simulink model "PID_Attitude_ver7_5"  (R2022a)
settings: Solver=FixedStepDiscrete  StartTime=0.0  StopTime=0.1  RelTol=1e-3
libraries: hdlsllib x1
settings Model: DataTypeOverride=Off  Creator=space  LastModifiedBy=space
settings OptimizationCC: BlockReduction=off  ConditionallyExecuteInputs=off  DefaultParameterBehavior=Inlined  InheritOutputTypeSmallerThanSingle=on
settings DebuggingCC: AlgebraicLoopMsg=error  SingleTaskRateTransMsg=error
settings HardwareCC: ProdBitPerPointer=32  ProdBitPerSizeT=32  ProdBitPerPtrDiffT=32  ProdLargestAtomicFloat=None  ProdIntDivRoundTo=Undefined  ProdEndianess=Unspecified  ProdWordSize=32  ProdHWDeviceType=ASIC/FPGA->ASIC/FPGA  TargetBitPerPointer=64  TargetBitPerSizeT=64  TargetBitPerPtrDiffT=64  TargetLongLongMode=on  TargetIntDivRoundTo=Zero  TargetEndianess=LittleEndian  TargetWordSize=64  TargetHWDeviceType=Custom Processor->MATLAB Host Computer  ProdEqTarget=off

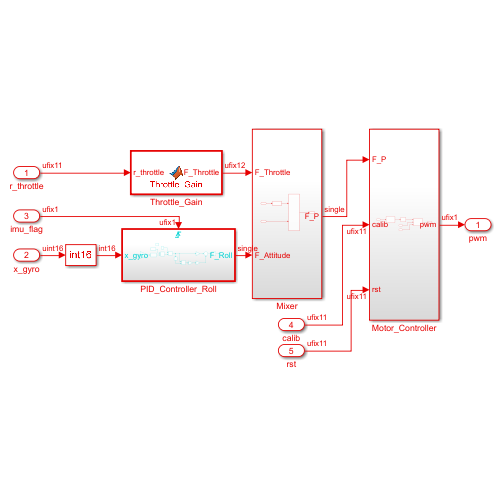
[thumbnail: Simulink's stored preview of the top-level diagram]
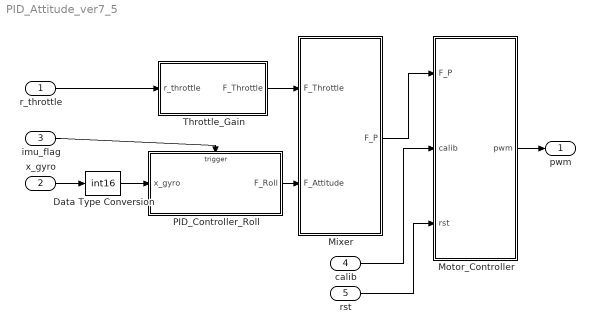
== system PID_Attitude_ver7_5 ==
  r_throttle : Inport  OutDataTypeStr=fixdt(0,11,0)
  x_gyro : Inport  Port=2  OutDataTypeStr=uint16
  imu_flag : Inport  Port=3  OutDataTypeStr=fixdt(0,1,0)
  calib : Inport  Port=4  OutDataTypeStr=fixdt(0,11,0)
  rst : Inport  Port=5  OutDataTypeStr=fixdt(0,11,0)
  Data Type Conversion : DataTypeConversion  OutDataTypeStr=int16  SaturateOnIntegerOverflow=off  RndMeth=Floor
  Mixer : Subsystem
  Motor_Controller : Subsystem
  PID_Controller_Roll : Subsystem
  Throttle_Gain : MATLAB Function  TreatAsAtomicUnit=on
  pwm : Outport  VectorParamsAs1DForOutWhenUnconnected=off
  wires:
  imu_flag/1 -> PID_Controller_Roll/Trigger
  Mixer/1(F_P) -> Motor_Controller/1(F_P)
  Motor_Controller/1(pwm) -> pwm/1
  rst/1 -> Motor_Controller/3(rst)
  r_throttle/1 -> Throttle_Gain/1(r_throttle)
  PID_Controller_Roll/1(F_Roll) -> Mixer/2(F_Attitude)
  Throttle_Gain/1(F_Throttle) -> Mixer/1(F_Throttle)
  x_gyro/1 -> Data Type Conversion/1
  Data Type Conversion/1 -> PID_Controller_Roll/1(x_gyro)
  calib/1 -> Motor_Controller/2(calib)

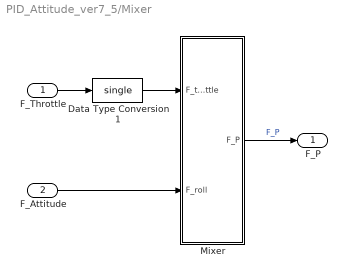
== system PID_Attitude_ver7_5/Mixer ==
  F_Throttle : Inport
  F_Attitude : Inport  Port=2
  Data Type Conversion1 : DataTypeConversion  OutDataTypeStr=single  SaturateOnIntegerOverflow=off  RndMeth=Floor
  Mixer : MATLAB Function  TreatAsAtomicUnit=on
  F_P : Outport
  wires:
  F_Throttle/1 -> Data Type Conversion1/1
  Mixer/1(F_P) -> F_P/1  "F_P"
  Data Type Conversion1/1 -> Mixer/1(F_throttle)
  F_Attitude/1 -> Mixer/2(F_roll)

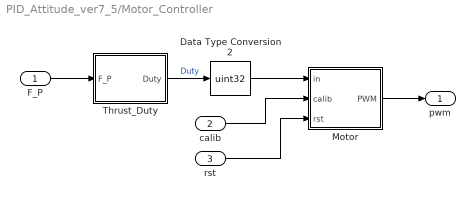
== system PID_Attitude_ver7_5/Motor_Controller ==
  F_P : Inport
  calib : Inport  Port=2  OutDataTypeStr=fixdt(0,11,0)
  rst : Inport  Port=3  OutDataTypeStr=fixdt(0,11,0)
  Data Type Conversion2 : DataTypeConversion  OutDataTypeStr=uint32  SaturateOnIntegerOverflow=off  RndMeth=Floor
  Motor : Subsystem
  Thrust_Duty : MATLAB Function  TreatAsAtomicUnit=on
  pwm : Outport
  wires:
  Thrust_Duty/1(Duty) -> Data Type Conversion2/1  "Duty"
  F_P/1 -> Thrust_Duty/1(F_P)
  Data Type Conversion2/1 -> Motor/1(in)
  calib/1 -> Motor/2(calib)
  rst/1 -> Motor/3(rst)
  Motor/1(PWM) -> pwm/1

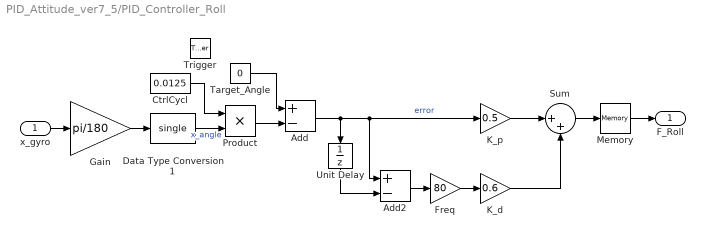
== system PID_Attitude_ver7_5/PID_Controller_Roll ==
  x_gyro : Inport
  Trigger : TriggerPort  VariantControl=(inherit)  PortDimensions=1
  Add : Sum  Inputs=+-
  Add2 : Sum  Inputs=+-
  CtrlCycl : Constant  Value=0.0125  VectorParams1D=off  OutDataTypeStr=single  SampleTime=-1
  Data Type Conversion1 : DataTypeConversion  OutDataTypeStr=single  SaturateOnIntegerOverflow=off  RndMeth=Floor
  Freq : Gain  Gain=80
  Gain : Gain  Gain=pi/180
  K_d : Gain  Gain=0.6
  K_p : Gain  Gain=0.5
  Memory : Memory  InheritSampleTime=on
  Product : Product
  Sum : Sum  Inputs=|++
  Target_Angle : Constant  Value=0  VectorParams1D=off  OutDataTypeStr=single  SampleTime=-1
  Unit Delay : UnitDelay  SampleTime=-1  HasFrameUpgradeWarning=on
  F_Roll : Outport  InitialOutput=0
  wires:
  Product/1 -> Add/2
  Add/1 -> K_p/1, Add2/1, Unit Delay/1  "error"
  Data Type Conversion1/1 -> Product/2  "x_angle"
  Add2/1 -> Freq/1
  x_gyro/1 -> Gain/1
  Target_Angle/1 -> Add/1
  Unit Delay/1 -> Add2/2
  K_d/1 -> Sum/2
  Freq/1 -> K_d/1
  CtrlCycl/1 -> Product/1
  Gain/1 -> Data Type Conversion1/1
  K_p/1 -> Sum/1
  Sum/1 -> Memory/1
  Memory/1 -> F_Roll/1

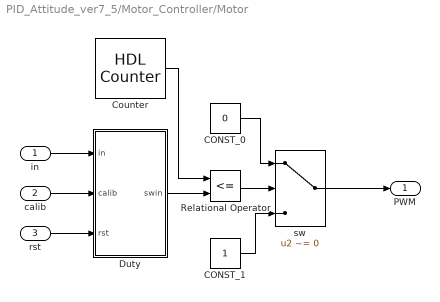
== system PID_Attitude_ver7_5/Motor_Controller/Motor ==
  in : Inport
  calib : Inport  Port=2
  rst : Inport  Port=3
  CONST_0 : Constant  Value=0  OutDataTypeStr=fixdt(0, 1, 0)  SampleTime=-1
  CONST_1 : Constant  OutDataTypeStr=fixdt(0, 1, 0)  SampleTime=-1
  Counter : hdlsllib/Sources/HDL Counter  CountType=Count limited  CountInit="fi(0,0,17,0,\"hex\",\"00\")"  CountStep="fi(0,0,17,0,\"hex\",\"01\")"  CountMax="fi(0,0,17,0,\"hex\",\"1e848\")"  CountFromType=Initial value  CountFrom="fi(0,0,17,0,\"hex\",\"00\")"  CountResetPort=off  CountLoadPort=off  CountEnbPort=off  CountDirPort=off  CountHitOutputPort=off  CountDataType=Unsigned  CountWordLen=17  CountFracLen=0  CountSampTime=50000000
  Duty : MATLAB Function  TreatAsAtomicUnit=on
  Relational Operator : RelationalOperator  Operator=<=  OutDataTypeStr=boolean  InputSameDT=off
  sw : Switch  Criteria=u2 ~= 0  Threshold=double(0)  OutDataTypeStr=fixdt(0, 1, 0)  SampleTime=-1  SaturateOnIntegerOverflow=off  InputSameDT=off
  PWM : Outport
  wires:
  Counter/1 -> Relational Operator/1
  rst/1 -> Duty/3(rst)
  Relational Operator/1 -> sw/2
  in/1 -> Duty/1(in)
  CONST_1/1 -> sw/3
  sw/1 -> PWM/1
  Duty/1(swin) -> Relational Operator/2
  CONST_0/1 -> sw/1
  calib/1 -> Duty/2(calib)

== matlab function PID_Attitude_ver7_5/Mixer/Mixer ==
  settings: fimath=fimath('RoundingMethod', 'Floor','OverflowAction', 'Wrap','ProductMode', 'FullPrecision', 'SumMode', 'FullPrecision')
  data: F_throttle input; F_P output; F_roll input
function F_P  = Mixer(F_throttle, F_roll)

if F_throttle == 0
    F_P = single(0);
else
    F_P = single(1/4 * (F_throttle + F_roll));
end

== matlab function PID_Attitude_ver7_5/Motor_Controller/Motor/Duty ==
  settings: fimath=fimath('RoundingMethod', 'Floor','OverflowAction', 'Wrap','ProductMode', 'FullPrecision', 'SumMode', 'FullPrecision')
  data: in input; swin output; calib input; rst input
function swin = Duty(in, calib, rst)

if rst > 1000
    %reset
    rst = 0x1E848u32;
    swin = rst;
    %swin = [rst; rst; rst; rst];
elseif calib > 1050
    %PWM -> MAX
    max = 0x1F4u32;
    swin = max;
    %swin = [max; max; max; max];
elseif calib == 1024
    %PWM -> MIN
    min = 0x130B0u32;
    swin = min;
    %swin = [min; min; min; min];
elseif calib < 1000
    %PWM -> thrust
    swin = in;
    %swin = [in(1); in(2); in(3); in(4)];
else
    err = 0x130B0u32;
    swin = err;
    %swin = [err; err; err; err];
end

== matlab function PID_Attitude_ver7_5/Motor_Controller/Thrust_Duty ==
  settings: fimath=fimath('RoundingMethod', 'Floor','OverflowAction', 'Wrap','ProductMode', 'FullPrecision', 'SumMode', 'FullPrecision')
  data: F_P input; Duty output single
function Duty = Thrust_Duty(F_P)

if F_P > 7
    Duty = single(17329);%7N以上の時出力85%に固定
elseif F_P <= 0
    Duty = single(78000);%0N以下のとき出力0%に固定
else
    Duty = -8215 * F_P + 69165;
end

== matlab function PID_Attitude_ver7_5/Throttle_Gain ==
  settings: fimath=fimath('RoundingMethod', 'Floor','OverflowAction', 'Wrap','ProductMode', 'FullPrecision', 'SumMode', 'FullPrecision')
  data: F_Throttle output; r_throttle input
function F_Throttle = Throttle_Gain(r_throttle)

F_Throttle = r_throttle / 56 - 44 / 7;
